simulink model "Modified_SEPIC_SI_Capacitor_Modification"  (R2019b)
settings: Solver=VariableStepAuto  StartTime=0.0  StopTime=2.0  RelTol=1e-3
libraries: powerlib x43, simulink x1
settings Model: Creator=jarir  LastModifiedBy=jarir

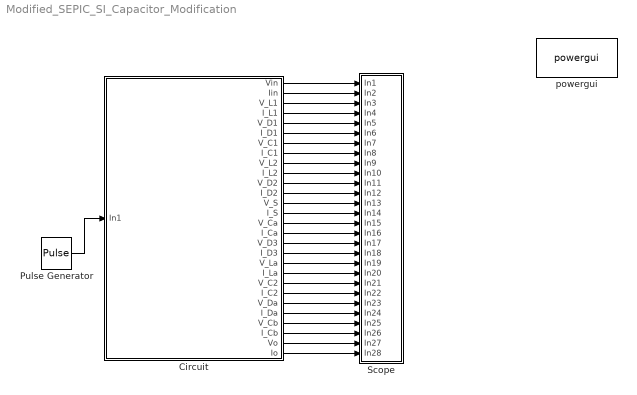
== system Modified_SEPIC_SI_Capacitor_Modification ==
  Circuit : Subsystem
  Pulse Generator : DiscretePulseGenerator  PulseType=Time based  Period=1/50000  PulseWidth=61.975
  Scope : Subsystem
  powergui : powerlib/powergui  Priority=1  SimulationMode=Continuous  SampleTime=50e-6  frequency=60  Iterations=50  frequencyindice=0  Pbase=100e6  ErrMax=1e-4  UnitsV=kV  UnitsW=MW  buscounter=0  FunctionMessages=off  echomessages=off  EnableUseOfTLC=off  CurrentSourceSwitches=off  DisableSnubberDevices=off  DisableRonSwitches=off  DisableVfSwitches=off  DisplayEquations=off  AutomaticDiscreteSolvers=off  SolverType=Tustin/Backward Euler (TBE)  Interpol=off  ExternalGateDelay=off  methode=off  Ts=100  x0status=blocks  SPID=on  SwTol=0  HookPort=off  NonlinearTolerance=1e-4  nMaxIteration=100  ContinueOnMaxIteration=off  RestoreLinks=warning  ResistiveCurrentMeasurement=off  Frange=[0:2:500]  Ylog=off  Xlog=on  ShowGrid=off  save=off  variable=ZData  structure=0  ZoomFFT=off  StartTime=0.0  cycles=1  DisplayStyle=1  fundamental=60  FreqAxis=off  MaxFrequency=1000  frequencyindicesteady=1  RmsSteady=1  display=off
      settings: SourceProductName=Simscape Electrical
  wires:
  Circuit/1(Vin) -> Scope/1(In1)
  Circuit/2(Iin) -> Scope/2(In2)
  Circuit/3(V_L1) -> Scope/3(In3)
  Circuit/4(I_L1) -> Scope/4(In4)
  Circuit/5(V_D1) -> Scope/5(In5)
  Circuit/6(I_D1) -> Scope/6(In6)
  Circuit/7(V_C1) -> Scope/7(In7)
  Circuit/8(I_C1) -> Scope/8(In8)
  Circuit/9(V_L2) -> Scope/9(In9)
  Circuit/10(I_L2) -> Scope/10(In10)
  Circuit/11(V_D2) -> Scope/11(In11)
  Circuit/12(I_D2) -> Scope/12(In12)
  Circuit/13(V_S) -> Scope/13(In13)
  Circuit/14(I_S) -> Scope/14(In14)
  Circuit/15(V_Ca) -> Scope/15(In15)
  Circuit/16(I_Ca) -> Scope/16(In16)
  Circuit/17(V_D3) -> Scope/17(In17)
  Circuit/18(I_D3) -> Scope/18(In18)
  Circuit/19(V_La) -> Scope/19(In19)
  Circuit/20(I_La) -> Scope/20(In20)
  Circuit/21(V_C2) -> Scope/21(In21)
  Circuit/22(I_C2) -> Scope/22(In22)
  Circuit/23(V_Da) -> Scope/23(In23)
  Circuit/24(I_Da) -> Scope/24(In24)
  Circuit/25(V_Cb) -> Scope/25(In25)
  Circuit/26(I_Cb) -> Scope/26(In26)
  Circuit/27(Vo) -> Scope/27(In27)
  Circuit/28(Io) -> Scope/28(In28)
  Pulse Generator/1 -> Circuit/1(In1)

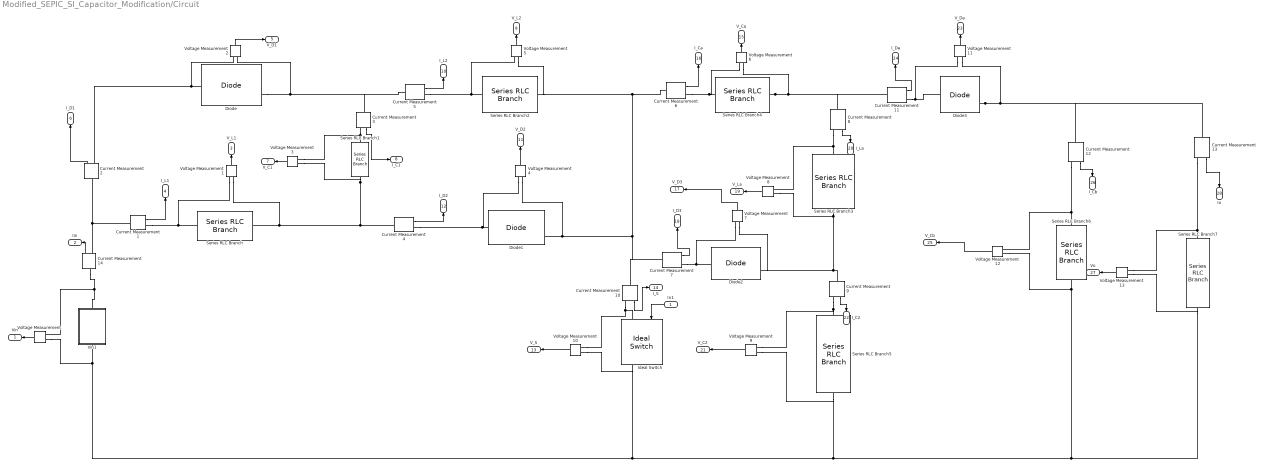
== system Modified_SEPIC_SI_Capacitor_Modification/Circuit ==
  In1 : Inport
  Current Measurement{1..14} (14 alike) : powerlib/Measurements/Current Measurement  PhasorSimulation=off  OutputType=Complex  PSBequivalent=0
      settings: SourceProductName=Simscape Electrical
  Diode{,1..3} (4 alike) : powerlib/Power Electronics/Diode  Ron=0.001  Lon=0  Vf=0.8  IC=0  UseSnubber=0  Rs=500  Cs=250e-9  Measurements=on
      settings: SourceProductName=Simscape Electrical
  Ideal Switch : powerlib/Power Electronics/Ideal Switch  Ron=0.001  Lon=0  IC=0  Rs=1e5  Cs=inf  Measurements=on
      settings: SourceProductName=Simscape Electrical
  Series RLC Branch : powerlib/Elements/Series RLC Branch  LConnTagsString=__new0  RConnTagsString=__new0  BranchType=L  Resistance=1  Inductance=500e-6  SetiL0=off  InitialCurrent=0  Capacitance=1e-6  Setx0=off  InitialVoltage=0  Measurements=None
      settings: SourceProductName=Simscape Electrical
  Series RLC Branch1 : powerlib/Elements/Series RLC Branch  LConnTagsString=__new0  RConnTagsString=__new0  BranchType=C  Resistance=1  Inductance=220e-6  SetiL0=off  InitialCurrent=0  Capacitance=470e-6  Setx0=off  InitialVoltage=0  Measurements=None
      settings: SourceProductName=Simscape Electrical
  Series RLC Branch2 : powerlib/Elements/Series RLC Branch  LConnTagsString=__new0  RConnTagsString=__new0  BranchType=L  Resistance=1  Inductance=500e-6  SetiL0=off  InitialCurrent=0  Capacitance=1e-6  Setx0=off  InitialVoltage=0  Measurements=None
      settings: SourceProductName=Simscape Electrical
  Series RLC Branch3 : powerlib/Elements/Series RLC Branch  LConnTagsString=__new0  RConnTagsString=__new0  BranchType=L  Resistance=1  Inductance=500e-6  SetiL0=off  InitialCurrent=0  Capacitance=1e-6  Setx0=off  InitialVoltage=0  Measurements=None
      settings: SourceProductName=Simscape Electrical
  Series RLC Branch4 : powerlib/Elements/Series RLC Branch  LConnTagsString=__new0  RConnTagsString=__new0  BranchType=C  Resistance=1  Inductance=220e-6  SetiL0=off  InitialCurrent=0  Capacitance=220e-6  Setx0=off  InitialVoltage=0  Measurements=None
      settings: SourceProductName=Simscape Electrical
  Series RLC Branch5 : powerlib/Elements/Series RLC Branch  LConnTagsString=__new0  RConnTagsString=__new0  BranchType=C  Resistance=1  Inductance=220e-6  SetiL0=off  InitialCurrent=0  Capacitance=220e-6  Setx0=off  InitialVoltage=0  Measurements=None
      settings: SourceProductName=Simscape Electrical
  Series RLC Branch6 : powerlib/Elements/Series RLC Branch  LConnTagsString=__new0  RConnTagsString=__new0  BranchType=C  Resistance=1  Inductance=220e-6  SetiL0=off  InitialCurrent=0  Capacitance=220e-6  Setx0=off  InitialVoltage=0  Measurements=None
      settings: SourceProductName=Simscape Electrical
  Series RLC Branch7 : powerlib/Elements/Series RLC Branch  LConnTagsString=__new0  RConnTagsString=__new0  BranchType=R  Resistance=320  Inductance=220e-6  SetiL0=off  InitialCurrent=0  Capacitance=220e-6  Setx0=off  InitialVoltage=0  Measurements=None
      settings: SourceProductName=Simscape Electrical
  Vin1 : Subsystem
  Voltage Measurement{,1..13} (14 alike) : powerlib/Measurements/Voltage Measurement  PhasorSimulation=off  OutputType=Complex  PSBequivalent=0
      settings: SourceProductName=Simscape Electrical
  Vin : Outport
  Iin : Outport  Port=2
  V_L1 : Outport  Port=3
  I_L1 : Outport  Port=4
  V_D1 : Outport  Port=5
  I_D1 : Outport  Port=6
  V_C1 : Outport  Port=7
  I_C1 : Outport  Port=8
  V_L2 : Outport  Port=9
  I_L2 : Outport  Port=10
  V_D2 : Outport  Port=11
  I_D2 : Outport  Port=12
  V_S : Outport  Port=13
  I_S : Outport  Port=14
  V_Ca : Outport  Port=15
  I_Ca : Outport  Port=16
  V_D3 : Outport  Port=17
  I_D3 : Outport  Port=18
  V_La : Outport  Port=19
  I_La : Outport  Port=20
  V_C2 : Outport  Port=21
  I_C2 : Outport  Port=22
  V_Da : Outport  Port=23
  I_Da : Outport  Port=24
  V_Cb : Outport  Port=25
  I_Cb : Outport  Port=26
  Vo : Outport  Port=27
  Io : Outport  Port=28
  wires:
  In1/1 -> Ideal Switch/1
  Voltage Measurement/1 -> Vin/1
  Voltage Measurement1/1 -> V_L1/1
  Current Measurement1/1 -> I_L1/1
  Voltage Measurement2/1 -> V_D1/1
  Current Measurement2/1 -> I_D1/1
  Voltage Measurement3/1 -> V_C1/1
  Current Measurement3/1 -> I_C1/1
  Voltage Measurement5/1 -> V_L2/1
  Current Measurement5/1 -> I_L2/1
  Voltage Measurement4/1 -> V_D2/1
  Current Measurement4/1 -> I_D2/1
  Voltage Measurement10/1 -> V_S/1
  Current Measurement10/1 -> I_S/1
  Voltage Measurement6/1 -> V_Ca/1
  Current Measurement6/1 -> I_Ca/1
  Voltage Measurement8/1 -> V_La/1
  Current Measurement8/1 -> I_La/1
  Voltage Measurement9/1 -> V_C2/1
  Current Measurement9/1 -> I_C2/1
  Voltage Measurement11/1 -> V_Da/1
  Current Measurement11/1 -> I_Da/1
  Voltage Measurement12/1 -> V_Cb/1
  Current Measurement12/1 -> I_Cb/1
  Voltage Measurement13/1 -> Vo/1
  Current Measurement13/1 -> Io/1
  Voltage Measurement7/1 -> V_D3/1
  Current Measurement7/1 -> I_D3/1
  Current Measurement14/1 -> Iin/1
  connections:
  Current Measurement1/LConn1 -- Current Measurement14/RConn1 -- Current Measurement2/LConn1
  Series RLC Branch1/RConn1 -- Voltage Measurement3/LConn2 -- Current Measurement4/LConn1 -- Voltage Measurement1/LConn2 -- Series RLC Branch/RConn1
  Current Measurement7/LConn1 -- Current Measurement10/LConn1 -- Current Measurement6/LConn1 -- Voltage Measurement5/LConn2 -- Series RLC Branch2/RConn1 -- Voltage Measurement4/LConn2 -- Diode1/RConn1
  Series RLC Branch2/LConn1 -- Current Measurement5/RConn1 -- Voltage Measurement5/LConn1
  Vin1/LConn1 -- Ideal Switch/RConn1 -- Voltage Measurement10/LConn2 -- Voltage Measurement9/LConn2 -- Series RLC Branch5/RConn1 -- Voltage Measurement13/LConn2 -- Series RLC Branch7/RConn1 -- Voltage Measurement12/LConn2 -- Series RLC Branch6/RConn1 -- Voltage Measurement/LConn2
  Series RLC Branch4/LConn1 -- Current Measurement11/LConn1 -- Current Measurement8/LConn1 -- Voltage Measurement6/LConn2
  Series RLC Branch3/LConn1 -- Current Measurement9/LConn1 -- Voltage Measurement7/LConn2 -- Diode2/RConn1 -- Voltage Measurement8/LConn1
  Diode3/RConn1 -- Current Measurement13/LConn1 -- Current Measurement12/LConn1 -- Voltage Measurement11/LConn2
  Current Measurement1/RConn1 -- Voltage Measurement1/LConn1 -- Series RLC Branch/LConn1
  Current Measurement2/RConn1 -- Voltage Measurement2/LConn1 -- Diode/LConn1
  Current Measurement3/RConn1 -- Voltage Measurement3/LConn1 -- Series RLC Branch1/LConn1
  Voltage Measurement4/LConn1 -- Current Measurement4/RConn1 -- Diode1/LConn1
  Voltage Measurement2/LConn2 -- Current Measurement5/LConn1 -- Current Measurement3/LConn1 -- Diode/RConn1
  Current Measurement6/RConn1 -- Voltage Measurement6/LConn1 -- Series RLC Branch4/RConn1
  Current Measurement7/RConn1 -- Voltage Measurement7/LConn1 -- Diode2/LConn1
  Series RLC Branch3/RConn1 -- Current Measurement8/RConn1 -- Voltage Measurement8/LConn2
  Current Measurement9/RConn1 -- Voltage Measurement9/LConn1 -- Series RLC Branch5/LConn1
  Current Measurement10/RConn1 -- Voltage Measurement10/LConn1 -- Ideal Switch/LConn1
  Current Measurement11/RConn1 -- Voltage Measurement11/LConn1 -- Diode3/LConn1
  Series RLC Branch6/LConn1 -- Current Measurement12/RConn1 -- Voltage Measurement12/LConn1
  Current Measurement13/RConn1 -- Voltage Measurement13/LConn1 -- Series RLC Branch7/LConn1
  Vin1/RConn1 -- Current Measurement14/LConn1 -- Voltage Measurement/LConn1

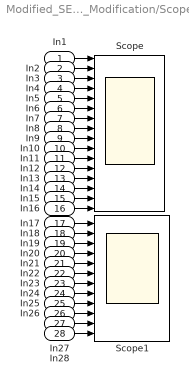
== system Modified_SEPIC_SI_Capacitor_Modification/Scope ==
  In1 : Inport
  In2 : Inport  Port=2
  In3 : Inport  Port=3
  In4 : Inport  Port=4
  In5 : Inport  Port=5
  In6 : Inport  Port=6
  In7 : Inport  Port=7
  In8 : Inport  Port=8
  In9 : Inport  Port=9
  In10 : Inport  Port=10
  In11 : Inport  Port=11
  In12 : Inport  Port=12
  In13 : Inport  Port=13
  In14 : Inport  Port=14
  In15 : Inport  Port=15
  In16 : Inport  Port=16
  In17 : Inport  Port=17
  In18 : Inport  Port=18
  In19 : Inport  Port=19
  In20 : Inport  Port=20
  In21 : Inport  Port=21
  In22 : Inport  Port=22
  In23 : Inport  Port=23
  In24 : Inport  Port=24
  In25 : Inport  Port=25
  In26 : Inport  Port=26
  In27 : Inport  Port=27
  In28 : Inport  Port=28
  Scope : Scope  NumInputPorts=16
  Scope1 : Scope  NumInputPorts=12
  wires:
  In18/1 -> Scope1/2
  In25/1 -> Scope1/9
  In17/1 -> Scope1/1
  In1/1 -> Scope/1
  In6/1 -> Scope/6
  In5/1 -> Scope/5
  In19/1 -> Scope1/3
  In22/1 -> Scope1/6
  In21/1 -> Scope1/5
  In20/1 -> Scope1/4
  In11/1 -> Scope/11
  In23/1 -> Scope1/7
  In24/1 -> Scope1/8
  In26/1 -> Scope1/10
  In2/1 -> Scope/2
  In28/1 -> Scope1/12
  In3/1 -> Scope/3
  In27/1 -> Scope1/11
  In4/1 -> Scope/4
  In8/1 -> Scope/8
  In9/1 -> Scope/9
  In7/1 -> Scope/7
  In10/1 -> Scope/10
  In12/1 -> Scope/12
  In13/1 -> Scope/13
  In14/1 -> Scope/14
  In16/1 -> Scope/16
  In15/1 -> Scope/15

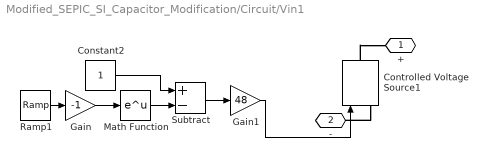
== system Modified_SEPIC_SI_Capacitor_Modification/Circuit/Vin1 ==
  Constant2 : Constant
  Controlled Voltage Source1 : powerlib/Electrical Sources/Controlled Voltage Source  Initialize=on  Source_Type=AC  Amplitude=0  Phase=0  Frequency=0  Measurements=None
      settings: SourceProductName=Simscape Electrical
  Gain : Gain  Gain=-1
  Gain1 : Gain  Gain=48
  Math Function : Math  SignedPower=off  SaturateOnIntegerOverflow=on
  Ramp1 : simulink/Sources/Ramp  slope=10  start=0  InitialOutput=0
  Subtract : Sum  Inputs=+-
  + : PMIOPort  Side=Right
  - : PMIOPort  Port=2  Side=Left
  wires:
  Gain1/1 -> Controlled Voltage Source1/1
  Constant2/1 -> Subtract/1
  Ramp1/1 -> Gain/1
  Math Function/1 -> Subtract/2
  Subtract/1 -> Gain1/1
  Gain/1 -> Math Function/1
  connections:
  Controlled Voltage Source1/RConn1 -- +/RConn1
  Controlled Voltage Source1/LConn1 -- -/RConn1
